simulink model "EnabledAndTriggeredSubSystem6Blocks"  (Simulink 7.6)
settings: Solver=ode45  StartTime=0.0  StopTime=10.0  RelTol=1e-3
settings Model: Creator=DominikC  LastModifiedBy=DominikC
settings DebuggingCC: FcnCallInpInsideContextMsg=Enable All

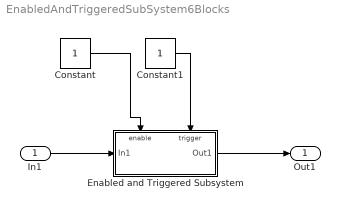
== system EnabledAndTriggeredSubSystem6Blocks ==
  In1 : Inport
  Constant : Constant
  Constant1 : Constant
  Enabled and Triggered Subsystem : Subsystem  TreatAsAtomicUnit=on
  Out1 : Outport
  wires:
  In1/1 -> Enabled and Triggered Subsystem/1(In1)
  Enabled and Triggered Subsystem/1(Out1) -> Out1/1
  Constant/1 -> Enabled and Triggered Subsystem/Enable
  Constant1/1 -> Enabled and Triggered Subsystem/Trigger

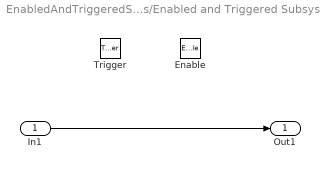
== system EnabledAndTriggeredSubSystem6Blocks/Enabled and Triggered Subsystem ==
  In1 : Inport
  Enable : EnablePort
  Trigger : TriggerPort
  Out1 : Outport
  wires:
  In1/1 -> Out1/1
